simulink model "dynamics"  (R2018a)
settings: Solver=VariableStepAuto  StartTime=0.0  StopTime=10.0  RelTol=1e-3
undefined symbols (not defined in the file): Cb, Cw, DiscIntNeverNeededParam, g, Ib, Iw, Km, l, lb, mb, mw
settings Model: Creator=henry  LastModifiedBy=henry

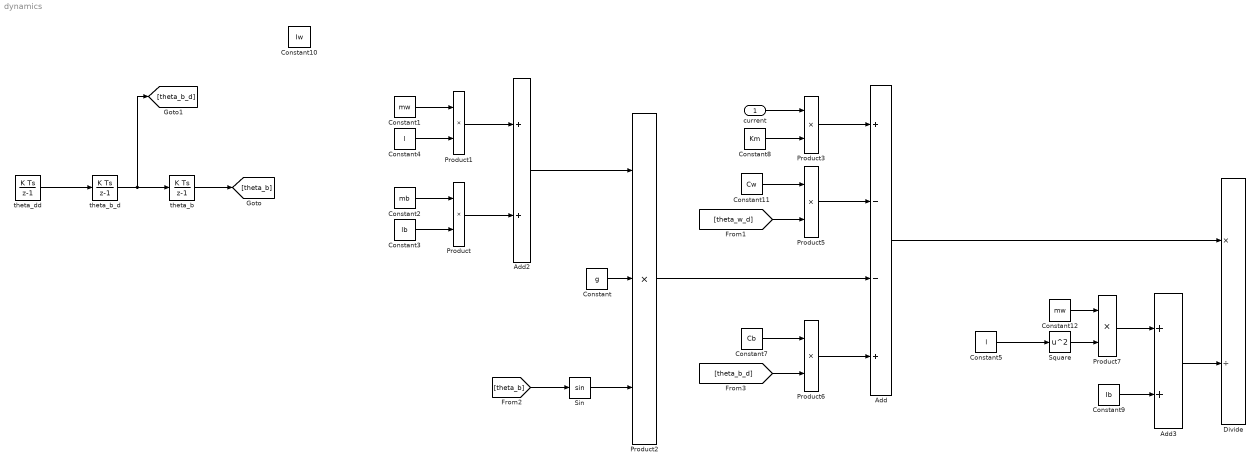
== system dynamics ==
  current : Inport
  Add : Sum  Inputs=+--+
  Add2 : Sum
  Add3 : Sum
  Constant : Constant  Value=g
  Constant1 : Constant  Value=mw
  Constant10 : Constant  Value=Iw
  Constant11 : Constant  Value=Cw
  Constant12 : Constant  Value=mw
  Constant2 : Constant  Value=mb
  Constant3 : Constant  Value=lb
  Constant4 : Constant  Value=l
  Constant5 : Constant  Value=l
  Constant7 : Constant  Value=Cb
  Constant8 : Constant  Value=Km
  Constant9 : Constant  Value=Ib
  Divide : Product  Inputs=*/
  Product{,1,3,5..7} (6 alike) : Product
  Product2 : Product  Inputs=3
  Sin : Trigonometry
  Square : Math  Operator=square  SaturateOnIntegerOverflow=on
  theta_b : DiscreteIntegrator  SampleTime=-1  ICPrevOutput=DiscIntNeverNeededParam  ICPrevScaledInput=DiscIntNeverNeededParam
  theta_b_d : DiscreteIntegrator  SampleTime=-1  ICPrevOutput=DiscIntNeverNeededParam  ICPrevScaledInput=DiscIntNeverNeededParam
  theta_dd : DiscreteIntegrator  SampleTime=-1  ICPrevOutput=DiscIntNeverNeededParam  ICPrevScaledInput=DiscIntNeverNeededParam
  wires:
  theta_dd/1 -> theta_b_d/1
  theta_b_d/1 -> [theta_b_d], theta_b/1
  Add/1 -> Divide/1
  Constant2/1 -> Product/1
  Constant3/1 -> Product/2
  Constant4/1 -> Product1/2
  Constant1/1 -> Product1/1
  Product1/1 -> Add2/1
  Product/1 -> Add2/2
  Add2/1 -> Product2/1
  Constant/1 -> Product2/2
  Sin/1 -> Product2/3
  theta_b/1 -> [theta_b]
  Constant11/1 -> Product5/1
  [theta_w_d] -> Product5/2
  current/1 -> Product3/1
  Constant8/1 -> Product3/2
  [theta_b] -> Sin/1
  Product2/1 -> Add/3
  Product3/1 -> Add/1
  Product5/1 -> Add/2
  Product6/1 -> Add/4
  [theta_b_d] -> Product6/2
  Constant7/1 -> Product6/1
  Constant5/1 -> Square/1
  Constant12/1 -> Product7/1
  Square/1 -> Product7/2
  Product7/1 -> Add3/1
  Constant9/1 -> Add3/2
  Add3/1 -> Divide/2
